simulink model "Priklad_3"  (R2022b)
settings: Solver=VariableStepAuto  StartTime=0.0  StopTime=150  RelTol=1e-3
settings Model: Creator=honza  LastModifiedBy=honza

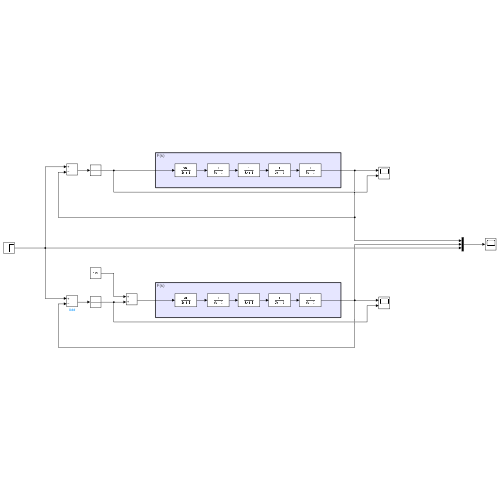
[thumbnail: Simulink's stored preview of the top-level diagram]
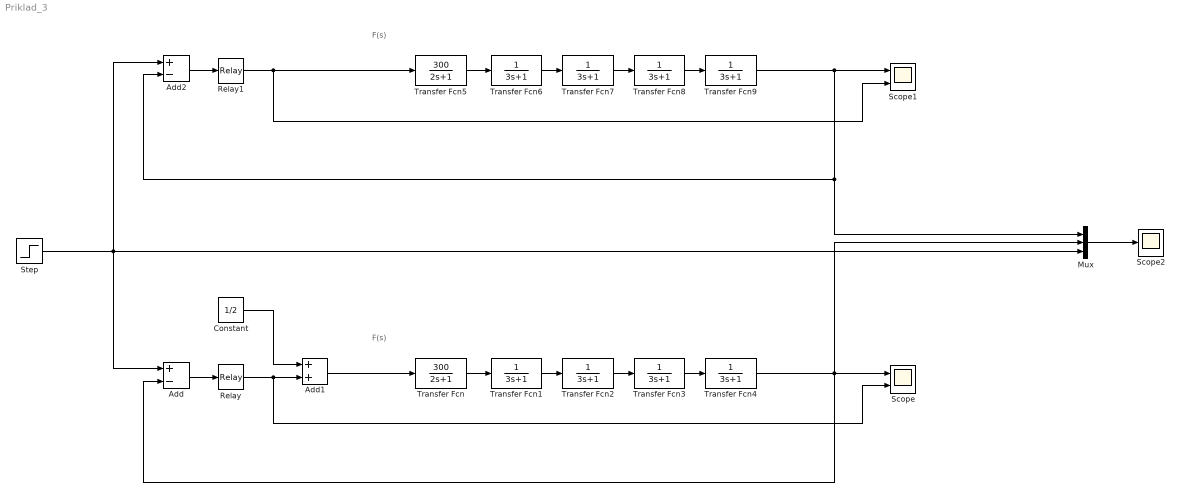
== system Priklad_3 ==
  note: F(s)
  note: F(s)
  Add : Sum  Inputs=+-
  Add1 : Sum
  Add2 : Sum  Inputs=+-
  Constant : Constant  Value=1/2
  Mux : Mux  Inputs=3
  Relay : Relay  OnSwitchValue=1/2  OffSwitchValue=0
  Relay1 : Relay  OnSwitchValue=1  OffSwitchValue=-1
  Scope : Scope  NumInputPorts=2
  Scope1 : Scope  NumInputPorts=2
  Scope2 : Scope
  Step : Step  Time=0  After=250  SampleTime=0
  Transfer Fcn : TransferFcn  Numerator=[300]  Denominator=[2 1]
  Transfer Fcn{1..4,6..9} (8 alike) : TransferFcn  Denominator=[3 1]
  Transfer Fcn5 : TransferFcn  Numerator=[300]  Denominator=[2 1]
  wires:
  Transfer Fcn1/1 -> Transfer Fcn2/1
  Add/1 -> Relay/1
  Transfer Fcn2/1 -> Transfer Fcn3/1
  Transfer Fcn4/1 -> Mux/2, Add/2, Scope/1
  Transfer Fcn3/1 -> Transfer Fcn4/1
  Transfer Fcn/1 -> Transfer Fcn1/1
  Add1/1 -> Transfer Fcn/1
  Relay/1 -> Add1/2, Scope/2
  Constant/1 -> Add1/1
  Relay1/1 -> Scope1/2, Transfer Fcn5/1
  Transfer Fcn5/1 -> Transfer Fcn6/1
  Transfer Fcn9/1 -> Mux/1, Add2/2, Scope1/1
  Transfer Fcn8/1 -> Transfer Fcn9/1
  Add2/1 -> Relay1/1
  Transfer Fcn7/1 -> Transfer Fcn8/1
  Transfer Fcn6/1 -> Transfer Fcn7/1
  Step/1 -> Add/1, Add2/1, Mux/3
  Mux/1 -> Scope2/1
